simulink model "Aufgabe_4_3_2__Zaehler_und_Stoppuhr"  (R2023b)
settings: Solver=ode3  StartTime=0.0  StopTime=20.0  FixedStep=0.01  RelTol=1e-3  EnableMultiTasking=on
settings Model: Creator=ASUS  LastModifiedBy=JCP
settings RTWCC: GPUComputeCapability=5.0

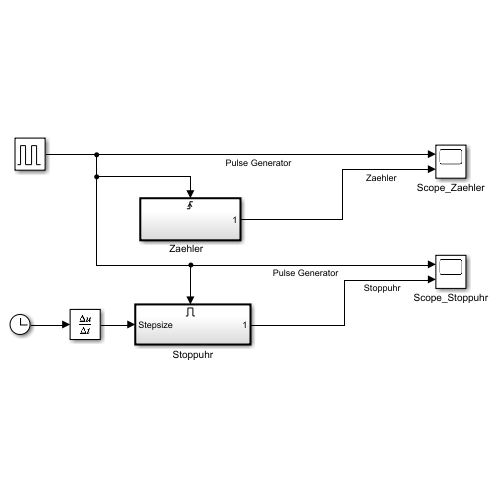
[thumbnail: Simulink's stored preview of the top-level diagram]
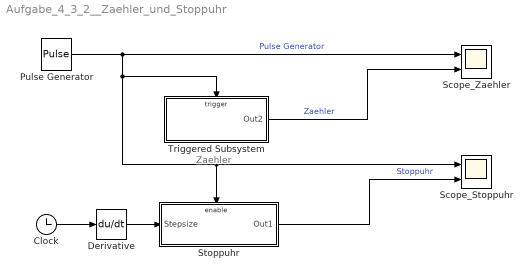
== system Aufgabe_4_3_2__Zaehler_und_Stoppuhr ==
  note: Zaehler
  Clock : Clock
  Derivative : Derivative
  Pulse Generator : DiscretePulseGenerator  PulseType=Time based  PulseWidth=50
  Scope_Stoppuhr : Scope  NumInputPorts=2
  Scope_Zaehler : Scope  NumInputPorts=2
  Stoppuhr : Subsystem  TreatAsAtomicUnit=on
  Triggered Subsystem : Subsystem  TreatAsAtomicUnit=on
  wires:
  Pulse Generator/1 -> Stoppuhr/Enable, Scope_Stoppuhr/1, Triggered Subsystem/Trigger, Scope_Zaehler/1  "Pulse Generator"
  Triggered Subsystem/1(Out2) -> Scope_Zaehler/2  "Zaehler"
  Derivative/1 -> Stoppuhr/1(Stepsize)
  Clock/1 -> Derivative/1
  Stoppuhr/1(Out1) -> Scope_Stoppuhr/2  "Stoppuhr"

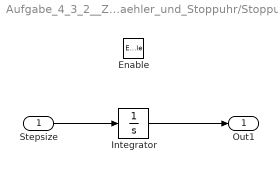
== system Aufgabe_4_3_2__Zaehler_und_Stoppuhr/Stoppuhr ==
  Stepsize : Inport
  Enable : EnablePort
  Integrator : Integrator
  Out1 : Outport
  wires:
  Stepsize/1 -> Integrator/1
  Integrator/1 -> Out1/1

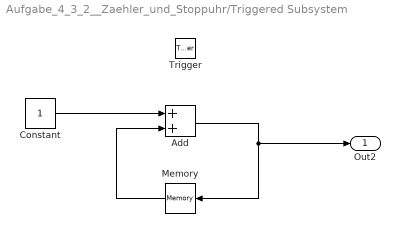
== system Aufgabe_4_3_2__Zaehler_und_Stoppuhr/Triggered Subsystem ==
  Trigger : TriggerPort  VariantControl=(inherit)
  Add : Sum
  Constant : Constant
  Memory : Memory  InheritSampleTime=on
  Out2 : Outport
  wires:
  Add/1 -> Memory/1, Out2/1
  Constant/1 -> Add/1
  Memory/1 -> Add/2
